simulink model "Synchr1"  (Simulink 4.00)
settings: Solver=ode45  StartTime=0.0  StopTime=1
InitFcn:
  | powericon('psbinitsys',bdroot);
libraries: powerlib2 x5
settings Model: SaveTime=off  SaveOutput=off  LimitDataPoints=off  BlockReductionOpt=off

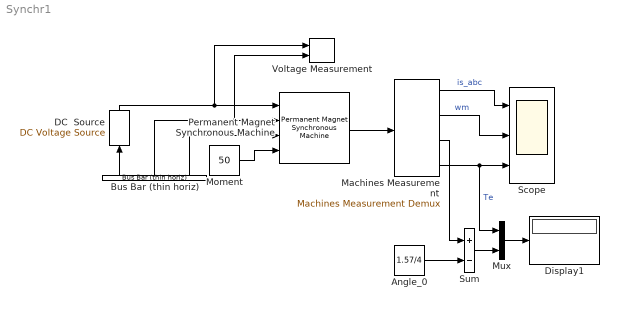
== system Synchr1 ==
  Angle_0 : Constant  Value=1.57/4
  Bus Bar (thin horiz) : powerlib2/Connectors/Bus Bar (thin horiz)  Tag=PoWeRsYsTeMbLoCk  Orientation=up  input=0  output=3  PSBOutputType=111111111111111111111111111111111111111111111111111111111111111111111111111111111111
  DC  Source : powerlib2/Electrical Sources/DC Voltage Source  Tag=PoWeRsYsTeMbLoCk  Description=source block  Orientation=up  V=100  mesure=None  PSBOutputType=1
  Display1 : Display
      settings: Format=short
  Machines Measurement : powerlib2/Machines/Machines Measurement Demux  machType=Permanent magnet synchronous  ssm1=on  ssm2=off  ssm3=on  ssm4=off  ssm5=on  ssm6=off  sm1=on  sm2=on  sm3=on  sm4=on  sm5=on  sm6=on  sm7=on  sm8=on  sm9=on  sm10=on  sm11=on  asm1=on  asm2=on  asm3=on  asm4=on  asm5=on  asm6=on  asm7=on  asm8=on  asm9=on  asm10=on  asm11=on  pmsm1=on  pmsm2=off  pmsm3=off  pmsm4=on  pmsm5=on  pmsm6=on  lastType=1
  Moment : Constant  Value=50
  Mux : Mux  Inputs=2
  Permanent Magnet Synchronous Machine : powerlib2/Machines/Permanent Magnet Synchronous Machine  Tag=PoWeRsYsTeMbLoCk  x1=2.8  x2=[8.5e-3, 2.5e-3]  x3=0.9  x4="[ 0.8e-3, 0,  4]"  PSBOutputType=0
  Scope : Scope  NumInputPorts=3
      settings: TimeRange=auto  YMin=-75~-50~-40  YMax=100~300~40  SaveToWorkspace=off  SaveName=ScopeData  MaxDataPoints=5000
  Sum : Sum  Inputs=+-  SaturateOnIntegerOverflow=on
  Voltage Measurement : powerlib2/Measurements/Voltage Measurement  Tag=PoWeRsYsTeMmEaSuReMeNt  PSBOutputType=0  PSBequivalent=1
  wires:
  Permanent Magnet Synchronous Machine/1 -> Machines Measurement/1
  Moment/1 -> Permanent Magnet Synchronous Machine/4
  Machines Measurement/2 -> Scope/2  "wm"
  Machines Measurement/1 -> Scope/1  "is_abc"
  Mux/1 -> Display1/1
  Machines Measurement/4 -> Mux/1, Scope/3  "Te"
  DC  Source/1 -> Permanent Magnet Synchronous Machine/1, Voltage Measurement/1
  Bus Bar (thin horiz)/1 -> DC  Source/1
  Bus Bar (thin horiz)/2 -> Permanent Magnet Synchronous Machine/2, Voltage Measurement/2
  Bus Bar (thin horiz)/3 -> Permanent Magnet Synchronous Machine/3
  Sum/1 -> Mux/2
  Machines Measurement/3 -> Sum/1
  Angle_0/1 -> Sum/2
